simulink model "desat_controller"  (R2018b)
settings: Solver=VariableStepAuto  StartTime=0.0  StopTime=1000  RelTol=1e-3
undefined symbols (not defined in the file or in its folder): fswParams, simParams
libraries: Environment_lib x1, aerolibutil x1, satelliteDynamics_lib x1, dspmtrx3 x1, dspstat3 x1, desat_controller_lib x1, rwa_allocation_lib x1
settings Model: Creator=sophiakim  LastModifiedBy=sophiakim

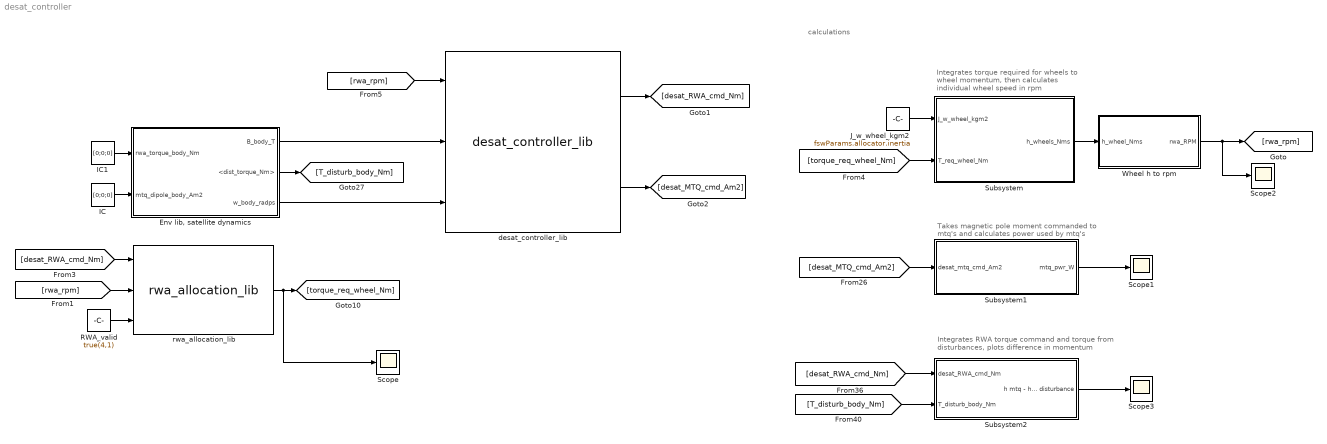
== system desat_controller ==
  note: Integrates RWA torque command and torque
      | from disturbances, plots difference in momentum
  note: Takes magnetic pole moment commanded
      | to mtq's and calculates power used by mtq's
  note: Integrates torque required for wheels
      | to wheel momentum, then calculates
      | individual wheel speed in rpm
  note: calculations
  "Env lib, satellite dynamics" : Subsystem
  IC : Constant  Value=[0;0;0]
  IC1 : Constant  Value=[0;0;0]
  J_w_wheel_kgm2 : Constant  Value=fswParams.allocator.inertia
  "RWA_valid " : Constant  Value=true(4,1)
  Scope{,1..3} (4 alike) : Scope
  Subsystem : Subsystem
  Subsystem1 : Subsystem
  Subsystem2 : Subsystem
  Wheel h to rpm : Subsystem
  desat_controller_lib : desat_controller_lib/desat_controller_lib  SystemSampleTime=-1
      link override Subsystem/Gain: Gain=[1 1 1 1]
      link override Subsystem1/Gain: Gain=fswParams.desatcontrollerParams.gain
  rwa_allocation_lib : rwa_allocation_lib/rwa_allocation_lib  SystemSampleTime=-1
  wires:
  desat_controller_lib/1 -> [desat_RWA_cmd_Nm]
  desat_controller_lib/2 -> [desat_MTQ_cmd_Am2]
  "RWA_valid "/1 -> rwa_allocation_lib/3
  [desat_RWA_cmd_Nm] -> rwa_allocation_lib/1
  J_w_wheel_kgm2/1 -> Subsystem/1(J_w_wheel_kgm2)
  [torque_req_wheel_Nm] -> Subsystem/2(T_req_wheel_Nm)
  [desat_MTQ_cmd_Am2] -> Subsystem1/1(desat_mtq_cmd_Am2)
  Subsystem1/1(mtq_pwr_W) -> Scope1/1
  [desat_RWA_cmd_Nm] -> Subsystem2/1(desat_RWA_cmd_Nm)
  [T_disturb_body_Nm] -> Subsystem2/2("T_disturb_body_Nm ")
  Subsystem2/1(h mtq - h disturbance) -> Scope3/1
  [rwa_rpm] -> rwa_allocation_lib/2
  [rwa_rpm] -> desat_controller_lib/1
  "Env lib, satellite dynamics"/1(B_body_T) -> desat_controller_lib/2
  "Env lib, satellite dynamics"/2(<dist_torque_Nm>) -> [T_disturb_body_Nm]
  IC1/1 -> "Env lib, satellite dynamics"/1(rwa_torque_body_Nm)
  IC/1 -> "Env lib, satellite dynamics"/2(mtq_dipole_body_Am2)
  Wheel h to rpm/1(rwa_RPM) -> Scope2/1, [rwa_rpm]
  Subsystem/1(h_wheels_Nms) -> Wheel h to rpm/1(h_wheel_Nms)
  rwa_allocation_lib/1 -> Scope/1, [torque_req_wheel_Nm]
  "Env lib, satellite dynamics"/3(w_body_radps) -> desat_controller_lib/3

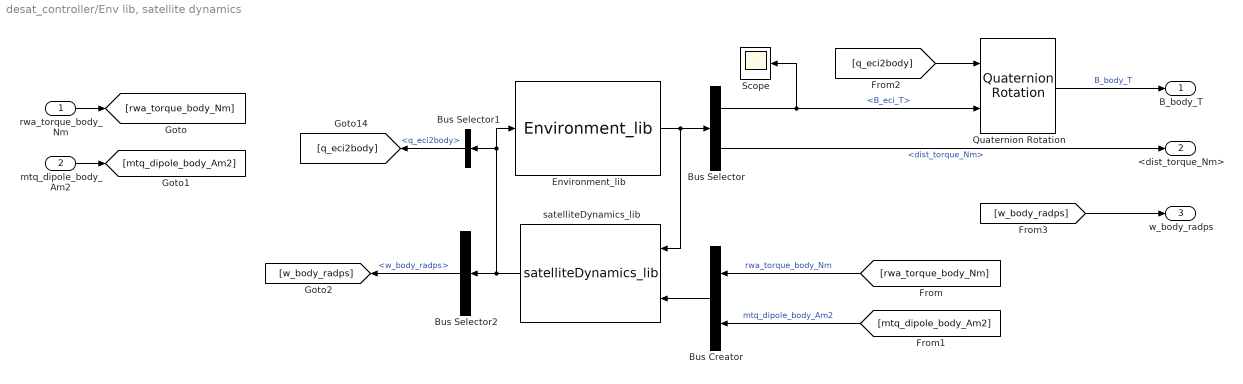
== system desat_controller/Env lib, satellite dynamics ==
  rwa_torque_body_Nm : Inport
  mtq_dipole_body_Am2 : Inport  Port=2
  Bus Creator : BusCreator  Inputs=2  OutDataTypeStr=Bus: actuator_control
  Bus Selector : BusSelector  OutputSignals=B_eci_T,dist_torque_Nm
  Bus Selector1 : BusSelector  OutputSignals=q_eci2body
  Bus Selector2 : BusSelector  OutputSignals=w_body_radps
  Environment_lib : Environment_lib/Environment_lib  SystemSampleTime=-1
  Quaternion Rotation : aerolibutil/Quaternion Rotation
  Scope : Scope
  satelliteDynamics_lib : satelliteDynamics_lib/satelliteDynamics_lib  SystemSampleTime=-1
  B_body_T : Outport
  <dist_torque_Nm> : Outport  Port=2
  w_body_radps : Outport  Port=3
  wires:
  [q_eci2body] -> Quaternion Rotation/1
  Bus Creator/1 -> satelliteDynamics_lib/2
  Bus Selector/1 -> Quaternion Rotation/2, Scope/1  "<B_eci_T>"
  Environment_lib/1 -> satelliteDynamics_lib/1, Bus Selector/1
  Quaternion Rotation/1 -> B_body_T/1  "B_body_T"
  satelliteDynamics_lib/1 -> Bus Selector2/1, Bus Selector1/1, Environment_lib/1
  [mtq_dipole_body_Am2] -> Bus Creator/2  "mtq_dipole_body_Am2"
  Bus Selector/2 -> <dist_torque_Nm>/1  "<dist_torque_Nm>"
  Bus Selector1/1 -> [q_eci2body]  "<q_eci2body>"
  [rwa_torque_body_Nm] -> Bus Creator/1  "rwa_torque_body_Nm"
  rwa_torque_body_Nm/1 -> [rwa_torque_body_Nm]
  mtq_dipole_body_Am2/1 -> [mtq_dipole_body_Am2]
  Bus Selector2/1 -> [w_body_radps]  "<w_body_radps>"
  [w_body_radps] -> w_body_radps/1

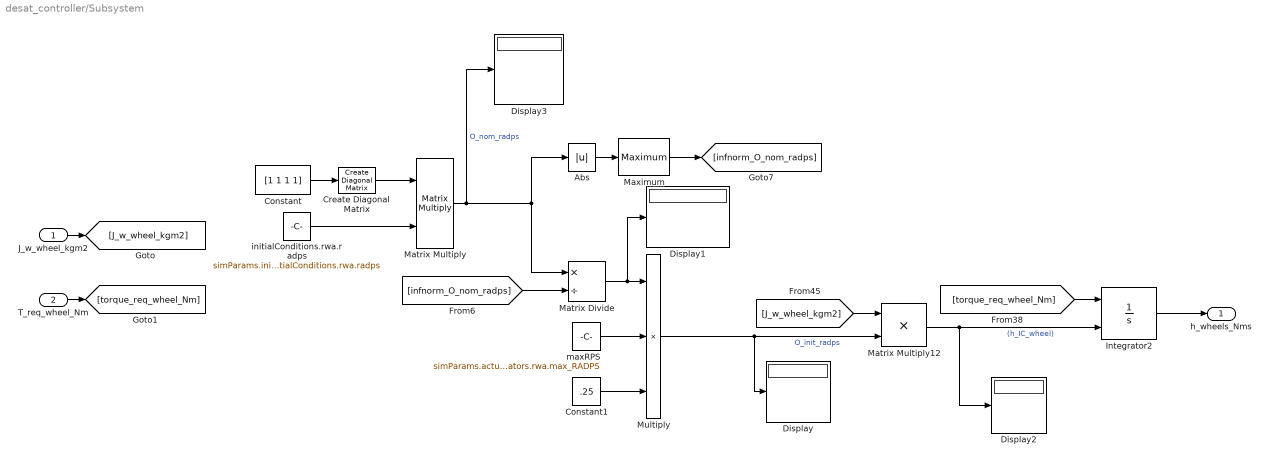
== system desat_controller/Subsystem ==
  J_w_wheel_kgm2 : Inport
  T_req_wheel_Nm : Inport  Port=2
  Abs : Abs
  Constant : Constant  Value=[1 1 1 1]
  Constant1 : Constant  Value=.25
  Create Diagonal Matrix : dspmtrx3/Create Diagonal Matrix
      settings: SourceProductName=DSP System Toolbox  SourceProductBaseCode=DS
  Display{,1..3} (4 alike) : Display
  Integrator2 : Integrator  InitialConditionSource=external
  Matrix Divide : Product  Inputs=*/
  Matrix Multiply : Product  Multiplication=Matrix(*)
  Matrix Multiply12 : Product
  Maximum : dspstat3/Maximum  operation=maximum  fcn=Value  indexBase=One  operateOver=Entire input  Dimension=1  InputProcessing=Columns as channels (frame based)  reset=None  roiEnable=off  roiType=Rectangles  roiPortion=Entire ROI  roiOutput=Individual statistics for each ROI  roiFlag=off  roundingMode=Floor  overflowMode=off  accumDataTypeStr=Inherit: Same as product output  accumLastDataTypeStr=Inherit: Same as product output
  Multiply : Product  Inputs=3
  initialConditions.rwa.radps : Constant  Value=simParams.initialConditions.rwa.radps
  maxRPS : Constant  Value=simParams.actuators.rwa.max_RADPS
  h_wheels_Nms : Outport
  wires:
  Integrator2/1 -> h_wheels_Nms/1
  Maximum/1 -> [infnorm_O_nom_radps]
  [infnorm_O_nom_radps] -> Matrix Divide/2
  Matrix Divide/1 -> Display1/1, Multiply/1
  Constant1/1 -> Multiply/3
  Matrix Multiply12/1 -> Display2/1, Integrator2/2  "(h_IC_wheel)"
  Multiply/1 -> Matrix Multiply12/2, Display/1  "O_init_radps"
  Constant/1 -> Create Diagonal Matrix/1
  maxRPS/1 -> Multiply/2
  [J_w_wheel_kgm2] -> Matrix Multiply12/1
  Create Diagonal Matrix/1 -> Matrix Multiply/1
  Matrix Multiply/1 -> Display3/1, Abs/1, Matrix Divide/1  "O_nom_radps"
  Abs/1 -> Maximum/1
  J_w_wheel_kgm2/1 -> [J_w_wheel_kgm2]
  T_req_wheel_Nm/1 -> [torque_req_wheel_Nm]
  initialConditions.rwa.radps/1 -> Matrix Multiply/2
  [torque_req_wheel_Nm] -> Integrator2/1

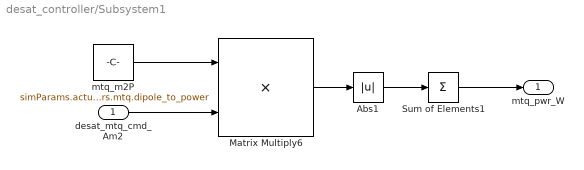
== system desat_controller/Subsystem1 ==
  desat_mtq_cmd_Am2 : Inport
  Abs1 : Abs
  Matrix Multiply6 : Product
  Sum of Elements1 : Sum  Inputs=+
  mtq_m2P : Constant  Value=simParams.actuators.mtq.dipole_to_power
  mtq_pwr_W : Outport
  wires:
  Sum of Elements1/1 -> mtq_pwr_W/1
  desat_mtq_cmd_Am2/1 -> Matrix Multiply6/2
  Matrix Multiply6/1 -> Abs1/1
  mtq_m2P/1 -> Matrix Multiply6/1
  Abs1/1 -> Sum of Elements1/1

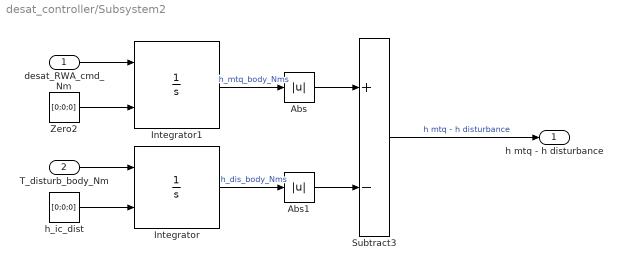
== system desat_controller/Subsystem2 ==
  desat_RWA_cmd_Nm : Inport
  "T_disturb_body_Nm " : Inport  Port=2
  Abs : Abs
  Abs1 : Abs
  Integrator : Integrator  InitialConditionSource=external
  Integrator1 : Integrator  InitialConditionSource=external
  Subtract3 : Sum  Inputs=+-
  Zero2 : Constant  Value=[0;0;0]  OutDataTypeStr=Inherit: Inherit via back propagation
  h_ic_dist : Constant  Value=[0;0;0]  OutDataTypeStr=Inherit: Inherit via back propagation
  h mtq - h disturbance : Outport
  wires:
  Subtract3/1 -> h mtq - h disturbance/1  "h mtq - h disturbance"
  Integrator/1 -> Abs1/1  "h_dis_body_Nms"
  Integrator1/1 -> Abs/1  "h_mtq_body_Nms"
  h_ic_dist/1 -> Integrator/2
  desat_RWA_cmd_Nm/1 -> Integrator1/1
  "T_disturb_body_Nm "/1 -> Integrator/1
  Zero2/1 -> Integrator1/2
  Abs/1 -> Subtract3/1
  Abs1/1 -> Subtract3/2

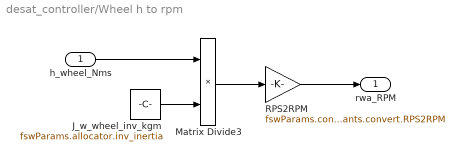
== system desat_controller/Wheel h to rpm ==
  h_wheel_Nms : Inport
  J_w_wheel_inv_kgm : Constant  Value=fswParams.allocator.inv_inertia
  Matrix Divide3 : Product  Inputs=**
  RPS2RPM : Gain  Gain=fswParams.constants.convert.RPS2RPM
  rwa_RPM : Outport
  wires:
  RPS2RPM/1 -> rwa_RPM/1
  Matrix Divide3/1 -> RPS2RPM/1
  h_wheel_Nms/1 -> Matrix Divide3/1
  J_w_wheel_inv_kgm/1 -> Matrix Divide3/2
